simulink model "exp03e03_pd"  (Simulink 8.9)
settings: Solver=FixedStepAuto  StartTime=0  StopTime=1  FixedStep=0.00442  RelTol=1e-10  EnableMultiTasking=on
values from neighbouring files (symbols this model uses):
  c1 = 2.94    [prelab03.m]
  k1 = 338.6    [prelab03.m]
  kd = 0.01    [prelab03.m]
  khw = 14732    [prelab03.m]
  kp = 0.08    [prelab03.m]
  kv = 0.005    [prelab03.m]
  m1 = mc1 + mw1    (= 2.778)    [prelab03.m]
libraries: simulink_need_slupdate x1, simulink_extras x1
settings Model: Creator=Giovani  LastModifiedBy=Gabriel
settings DataIOCC: LimitDataPoints=off
settings OptimizationCC: ExpressionDepthLimit=2147483647
settings DebuggingCC: SolverPrmCheckMsg=warning
settings GRTTargetCC: GeneratePreprocessorConditionals=Use local settings

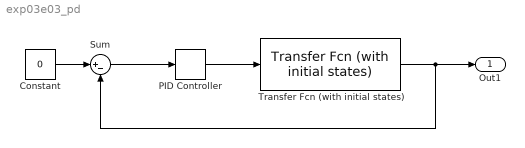
== system exp03e03_pd ==
  Constant : Constant  Value=0
  PID Controller : simulink_need_slupdate/PID Controller  P=kp  I=0  D=kd
      settings: SourceProductName=Simulink
  Sum : Sum  Inputs=|+-
  Transfer Fcn (with initial states) : simulink_extras/Additional Linear/Transfer Fcn (with initial states)  N=[khw]  D=[m1 (c1+khw*kv) k1]  X0=0
  Out1 : Outport
  wires:
  Sum/1 -> PID Controller/1
  PID Controller/1 -> Transfer Fcn (with initial states)/1
  Constant/1 -> Sum/1
  Transfer Fcn (with initial states)/1 -> Sum/2, Out1/1
